simulink model "ProjetoFinalControladorPIDnaolinear (1)"  (R2021a)
settings: Solver=ode4  StartTime=0.0  StopTime=50  FixedStep=1e-3  RelTol=1e-3  EnableMultiTasking=on
settings Model: Creator=Rafael  LastModifiedBy=joaom
settings SolverCC: AlgebraicLoopSolver=TrustRegion
settings DataIOCC: ReturnWorkspaceOutputs=off
settings OptimizationCC: LifeSpan=inf
settings DebuggingCC: SFUnexpectedBacktrackingDiag=warning  SFNoUnconditionalDefaultTransitionDiag=warning  SFMachineParentedDataDiag=warning  ArithmeticOperatorsInVariantConditions=warning
settings SFSimCC: SimUseLocalCustomCode=off  CustomCodeUndefinedFunction=UseInterfaceOnly
settings RTWCC: RTWUseLocalCustomCode=off
settings CodeAppCC: StateflowObjectComments=on
settings GRTTargetCC: TargetLangStandard=C89/C90 (ANSI)
settings ConfigComp: CovMetricSettings=dw  CovSaveCumulativeToWorkspaceVar=on  CovSaveSingleToWorkspaceVar=on  CovExternalEMLEnable=off

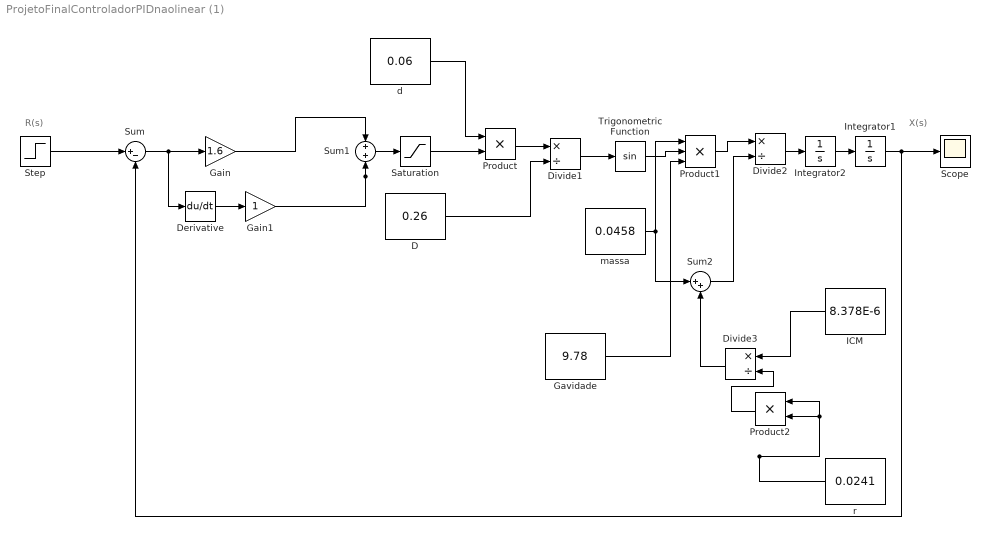
== system ProjetoFinalControladorPIDnaolinear (1) ==
  note: X(s)
  note: R(s)
  D : Constant  Value=0.26
  Derivative : Derivative
  Divide1 : Product  Inputs=*/
  Divide2 : Product  Inputs=*/
  Divide3 : Product  Inputs=*/
  Gain : Gain  Gain=1.6
  Gain1 : Gain
  Gavidade : Constant  Value=9.78
  ICM : Constant  Value=8.378E-6
  Integrator1 : Integrator
  Integrator2 : Integrator
  Product : Product
  Product1 : Product  Inputs=3
  Product2 : Product
  Saturation : Saturate  UpperLimit=0.785  LowerLimit=-0.785
  Scope : Scope
  Step : Step  Time=0  SampleTime=0
  Sum : Sum  Inputs=|+-
  Sum1 : Sum
  Sum2 : Sum  Inputs=|++
  Trigonometric Function : Trigonometry
  d : Constant  Value=0.06
  massa : Constant  Value=0.0458
  r : Constant  Value=0.0241
  wires:
  Step/1 -> Sum/1
  Integrator1/1 -> Sum/2, Scope/1
  Sum1/1 -> Saturation/1
  Integrator2/1 -> Integrator1/1
  Divide1/1 -> Trigonometric Function/1
  d/1 -> Product/1
  Saturation/1 -> Product/2
  Product/1 -> Divide1/1
  D/1 -> Divide1/2
  Trigonometric Function/1 -> Product1/2
  massa/1 -> Product1/1, Sum2/1
  Gavidade/1 -> Product1/3
  Product1/1 -> Divide2/1
  Sum2/1 -> Divide2/2
  Divide2/1 -> Integrator2/1
  Divide3/1 -> Sum2/2
  ICM/1 -> Divide3/1
  Product2/1 -> Divide3/2
  r/1 -> Product2/2, Product2/1
  Sum/1 -> Derivative/1, Gain/1
  Derivative/1 -> Gain1/1
  Gain1/1 -> Sum1/2
  Gain/1 -> Sum1/1
